simulink model "PVarray_normal"  (R2021a)
settings: Solver=VariableStepAuto  StartTime=0.0  StopTime=80  MaxStep=0.1  RelTol=1e-3
libraries: spsDiodeLib x15, spsPVArrayLib x12, spsControlledVoltageSourceLib x1, spsCurrentMeasurementLib x1, simulink x1, spsVoltageMeasurementLib x1, spspowerguiLib x1
settings Model: Creator=Lenovo  LastModifiedBy=Lenovo

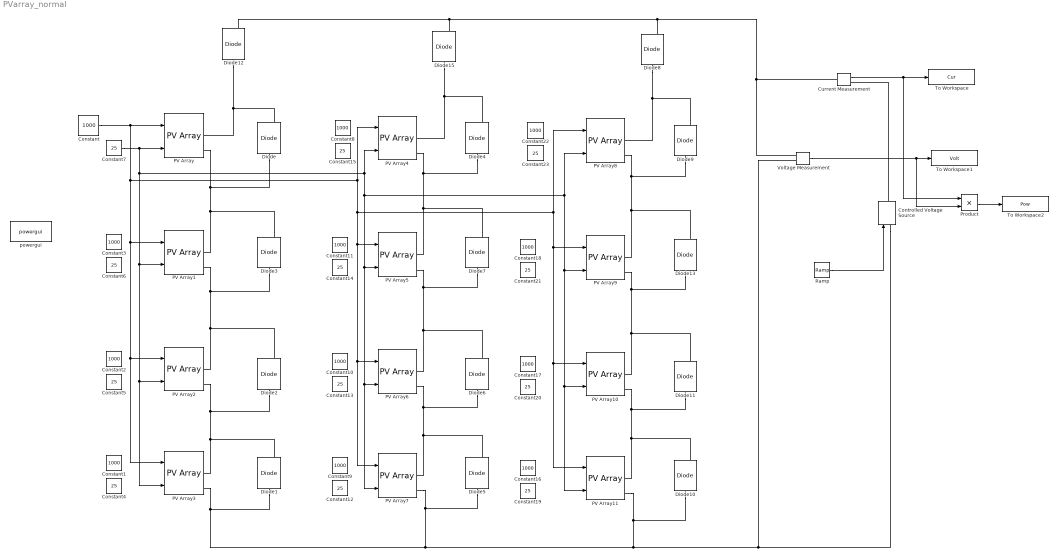
== system PVarray_normal ==
  Constant{,1..3,8..11,16..18,22} (12 alike) : Constant  Value=1000
  Constant{4..7,12..15,19..21,23} (12 alike) : Constant  Value=25
  Controlled Voltage Source : spsControlledVoltageSourceLib/Controlled Voltage Source  Initialize=on  Source_Type=AC  Amplitude=0  Phase=0  Frequency=0  Measurements=None
  Current Measurement : spsCurrentMeasurementLib/Current Measurement  PhasorSimulation=off  OutputType=Complex  PSBequivalent=0
  Diode{,1..13,15} (15 alike) : spsDiodeLib/Diode  Ron=0.001  Lon=0  Vf=0.8  IC=0  UseSnubber=0  Rs=500  Cs=250e-9  Measurements=on
  PV Array{,1..11} (12 alike) : spsPVArrayLib/PV Array  Npar=1  Nser=1  PlotType=array @ 1000 W/m2 & specified temperatures  S_vec="[ 1000  500  100 ]"  Temp_C_vec="[ 45 25  ]"  ModuleName=User-defined  PlotWhenSelected=off  Pm=79.92  Ncell=36  Voc=21.6  Isc=4.89  Vm=18  Im=4.44  beta_Voc_pc=-0.34  alpha_Isc_pc=0.045  beta_Voc=-0.07344  alpha_Isc=0.0022005  IL=4.9034  I0=7.7859e-11  nI=0.94142  Rsh=76.2104  Rs=0.20928  RobustModel=off  RobustCellTemperature=313.3991  BAL=on  Tc=1e-6  Tfilter=5e-5
  Product : Product
  Ramp : simulink/Sources/Ramp  slope=1  start=0  InitialOutput=0
  To Workspace : ToWorkspace  VariableName=Cur  SaveFormat=Timeseries  SampleTime=-1
  To Workspace1 : ToWorkspace  VariableName=Volt  SaveFormat=Timeseries  SampleTime=-1
  To Workspace2 : ToWorkspace  VariableName=Pow  SaveFormat=Timeseries  SampleTime=-1
  Voltage Measurement : spsVoltageMeasurementLib/Voltage Measurement  PhasorSimulation=off  OutputType=Complex  PSBequivalent=0
  powergui : spspowerguiLib/powergui  Priority=1  SimulationMode=Continuous  SampleTime=50e-6  frequency=60  Iterations=50  frequencyindice=0  Pbase=100e6  ErrMax=1e-4  UnitsV=kV  UnitsW=MW  buscounter=0  FunctionMessages=off  echomessages=off  EnableUseOfTLC=off  CurrentSourceSwitches=off  DisableSnubberDevices=off  DisableRonSwitches=off  DisableVfSwitches=off  DisplayEquations=off  AutomaticDiscreteSolvers=off  SolverType=Tustin/Backward Euler (TBE)  Interpol=off  ExternalGateDelay=off  methode=off  Ts=100  x0status=blocks  SPID=on  SwTol=0  HookPort=off  NonlinearTolerance=1e-4  nMaxIteration=100  ContinueOnMaxIteration=off  RestoreLinks=warning  ResistiveCurrentMeasurement=off  Frange=[0:2:500]  Ylog=off  Xlog=on  ShowGrid=off  save=off  variable=ZData  structure=0  ZoomFFT=off  StartTime=0.0  cycles=1  DisplayStyle=1  fundamental=60  FreqAxis=off  MaxFrequency=1000  frequencyindicesteady=1  RmsSteady=1  display=off
  wires:
  Ramp/1 -> Controlled Voltage Source/1
  Current Measurement/1 -> Product/1, To Workspace/1
  Voltage Measurement/1 -> Product/2, To Workspace1/1
  Product/1 -> To Workspace2/1
  Constant7/1 -> PV Array3/2, PV Array2/2, PV Array1/2, PV Array11/2, PV Array10/2, PV Array9/2, PV Array8/2, PV Array5/2, PV Array7/2, PV Array6/2, PV Array4/2, PV Array/2
  Constant/1 -> PV Array/1, PV Array1/1, PV Array2/1, PV Array3/1, PV Array9/1, PV Array10/1, PV Array11/1, PV Array8/1, PV Array5/1, PV Array6/1, PV Array7/1, PV Array4/1
  connections:
  Diode12/LConn1 -- Diode/RConn1 -- PV Array/RConn1
  Diode15/LConn1 -- Diode4/RConn1 -- PV Array4/RConn1
  PV Array4/RConn2 -- Diode4/LConn1 -- Diode7/RConn1 -- PV Array5/RConn1
  PV Array5/RConn2 -- Diode7/LConn1 -- Diode6/RConn1 -- PV Array6/RConn1
  PV Array6/RConn2 -- Diode6/LConn1 -- Diode5/RConn1 -- PV Array7/RConn1
  Current Measurement/LConn1 -- Diode8/RConn1 -- Diode12/RConn1 -- Diode15/RConn1 -- Voltage Measurement/LConn1
  Diode1/LConn1 -- PV Array3/RConn2 -- Diode5/LConn1 -- PV Array7/RConn2 -- Diode10/LConn1 -- PV Array11/RConn2 -- Controlled Voltage Source/LConn1 -- Voltage Measurement/LConn2
  Controlled Voltage Source/RConn1 -- Current Measurement/RConn1
  PV Array11/RConn1 -- Diode10/RConn1 -- PV Array10/RConn2 -- Diode11/LConn1
  PV Array8/RConn1 -- Diode8/LConn1 -- Diode9/RConn1
  PV Array10/RConn1 -- PV Array9/RConn2 -- Diode13/LConn1 -- Diode11/RConn1
  PV Array9/RConn1 -- PV Array8/RConn2 -- Diode9/LConn1 -- Diode13/RConn1
  Diode3/RConn1 -- PV Array1/RConn1 -- PV Array/RConn2 -- Diode/LConn1
  Diode2/LConn1 -- PV Array2/RConn2 -- Diode1/RConn1 -- PV Array3/RConn1
  Diode3/LConn1 -- PV Array1/RConn2 -- Diode2/RConn1 -- PV Array2/RConn1
